simulink model "rect_1_diode"  (Simulink 7.9)
settings: Solver=ode23tb  StartTime=0.0  StopTime=1  MaxStep=1e-5  RelTol=1e-5
libraries: powerlib x8
settings Model: Creator=User  LastModifiedBy=User
settings DataIOCC: SignalLoggingName=sigsOut
settings DebuggingCC: SaveWithParameterizedLinksMsg=none  SignalResolutionControl=TryResolveAllWithWarning  SolverPrmCheckMsg=none  MultiTaskDSMMsg=warning  MultiTaskCondExecSysMsg=none  StrictBusMsg=None
settings HardwareCC: TargetUnknown=on
settings RTWCC: IncludeERTFirstTime=on
settings GRTTargetCC: CombineOutputUpdateFcns=off  GRTInterface=on

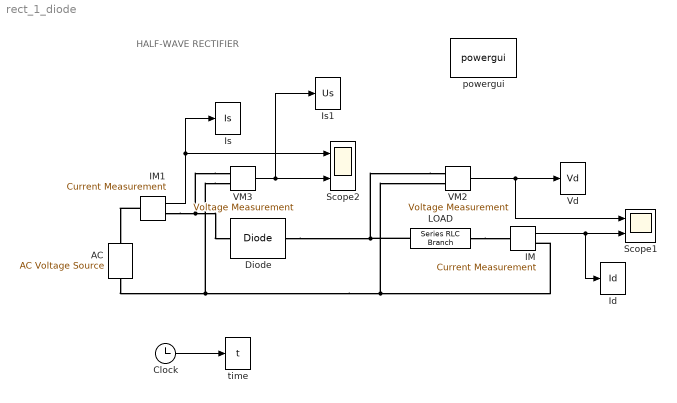
== system rect_1_diode ==
  note: HALF-WAVE RECTIFIER
  "AC " : powerlib/Electrical Sources/AC Voltage Source  Description=source block  Amplitude=220*sqrt(2)  Phase=0  Frequency=50  SampleTime=0  Measurements=None
      settings: AttributesFormatString=\n
  Clock : Clock
  Diode : powerlib/Power Electronics/Diode  Ron=0.001  Lon=0  Vf=0.8  IC=0  UseSnubber=off  Rs=1e4  Cs=inf  Measurements=off
  IM : powerlib/Measurements/Current Measurement  Tag=PoWeRsYsTeMmEaSuReMeNt  PhasorSimulation=off  OutputType=Magnitude  PSBequivalent=0
  IM1 : powerlib/Measurements/Current Measurement  Tag=PoWeRsYsTeMmEaSuReMeNt  PhasorSimulation=off  OutputType=Magnitude  PSBequivalent=0
  Id : ToWorkspace  VariableName=Id  SampleTime=-1
  Is : ToWorkspace  VariableName=Is  SampleTime=-1
  Is1 : ToWorkspace  VariableName=Us  SampleTime=-1
  LOAD : powerlib/Elements/Series RLC Branch  LConnTagsString=__new0  RConnTagsString=__new0  BranchType=RL  Resistance=10  Inductance=50e-3  SetiL0=off  InitialCurrent=0  Capacitance=inf  Setx0=off  InitialVoltage=0  Measurements=None
  Scope1 : Scope  NumInputPorts=2
      settings: YMin=-125~-1  YMax=100~7
  Scope2 : Scope  NumInputPorts=2
      settings: YMin=-5~-5  YMax=5~5  SaveName=ScopeData2
  VM2 : powerlib/Measurements/Voltage Measurement  PhasorSimulation=off  OutputType=Complex  PSBequivalent=0
  VM3 : powerlib/Measurements/Voltage Measurement  PhasorSimulation=off  OutputType=Complex  PSBequivalent=0
  Vd : ToWorkspace  VariableName=Vd  SampleTime=-1
  powergui : powerlib/powergui  Priority=1  SimulationMode=Continuous  SolverType=Tustin  SampleTime=50e-6  frequency=60  SPID=off  DisableSnubberDevices=off  DisableRonSwitches=off  DisableVfSwitches=off  SwTol=0  Interpol=off  DisplayEquations=off  FunctionMessages=off  frequencyindice=50  Pbase=100e6  ErrMax=1e-4  Iterations=50  UnitsV=kV  UnitsW=MW  echomessages=off  HookPort=off  EnableUseOfTLC=off  x0status=blocks  RestoreLinks=warning  ResistiveCurrentMeasurement=off  Ylog=off  Xlog=on  ShowGrid=off  save=off  variable=ZData  ZoomFFT=off  StartTime=0.0  cycles=1  DisplayStyle=1  FreqAxis=off  MaxFrequency=1000  frequencyindicesteady=1  display=off  methode=off
  time : ToWorkspace  VariableName=t  SampleTime=-1
  wires:
  IM/1 -> Scope1/2, Id/1
  VM2/1 -> Scope1/1, Vd/1
  IM1/1 -> Is/1, Scope2/1
  Clock/1 -> time/1
  VM3/1 -> Scope2/2, Is1/1
  connections:
  IM1/LConn1 -- "AC "/RConn1
  VM3/LConn2 -- "AC "/LConn1 -- IM/RConn1 -- VM2/LConn2
  VM2/LConn1 -- LOAD/LConn1 -- Diode/RConn1
  LOAD/RConn1 -- IM/LConn1
  VM3/LConn1 -- IM1/RConn1 -- Diode/LConn1
